simulink model "rapros_quadrotor_PID"  (R2013a)
settings: Solver=ode45  StartTime=0.0  StopTime=350  RelTol=1e-3
InitFcn:
  | parameters
values from neighbouring files (symbols this model uses):
  MATRIX = [-0.25 0 0.5 0.25 ... (first row only)    [parameters.m]
  X0 = [0;0;0;0;0;0;0;0;0;0;0;0]    [parameters.m]
libraries: instrumentlib x2, simulink x1
settings Model: Creator=root  LastModifiedBy=root
settings SolverCC: MaxConsecutiveMinStep=50000  AutoInsertRateTranBlk=on
settings DataIOCC: SignalLoggingSaveFormat=ModelDataLogs  SaveOutput=off  SaveTime=off
settings OptimizationCC: InlineParams=on  InlineInvariantSignals=on  StateBitsets=on  DataBitsets=on  UseTempVars=on  ZeroExternalMemoryAtStartup=off  ZeroInternalMemoryAtStartup=off  NoFixptDivByZeroProtection=on  OptimizeModelRefInitCode=on  LifeSpan=1
settings DebuggingCC: MultiTaskDSMMsg=warning  MultiTaskCondExecSysMsg=none  StrictBusMsg=None
settings HardwareCC: ProdIntDivRoundTo=Floor  ProdEndianess=LittleEndian  ProdHWDeviceType=Generic->Custom
settings RTWCC: SystemTargetFile=ert.tlc  TLCOptions=-p0  GenCodeOnly=on  TemplateMakefile=ert_default_tmf  Description=Embedded Coder  GenerateReport=on  RTWVerbose=off  ProcessScript=ert_make_rtw_hook  IncludeHyperlinkInReport=on  LaunchReport=on  IncludeERTFirstTime=on
settings CodeAppCC: ForceParamTrailComments=on  IgnoreCustomStorageClasses=off  SimulinkDataObjDesc=on  CustomSymbolStrGlobalVar=rt$N$M  CustomSymbolStrType=$N$M  CustomSymbolStrFcn=$N$M$F  CustomSymbolStrMacro=$N$M  InsertBlockDesc=on
settings ERTTargetCC: CodeReplacementLibrary=None  IncludeMdlTerminateFcn=off  SuppressErrorStatus=on  SupportAbsoluteTime=off  SupportNonFinite=off  SupportComplex=off  PurelyIntegerCode=on  RootIOFormat=Structure reference  ERTCustomFileTemplate=example_file_process.tlc

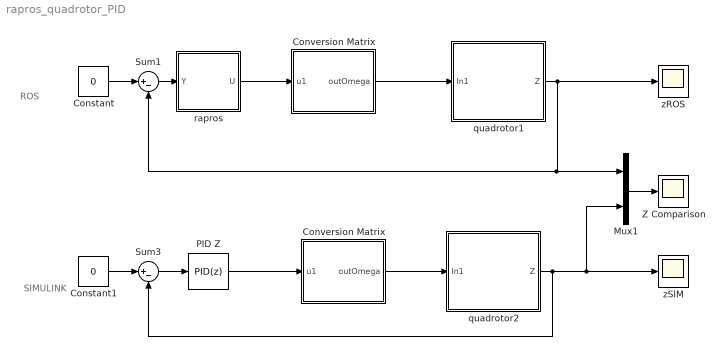
== system rapros_quadrotor_PID ==
  note: ROS
  note: SIMULINK
  Constant : Constant  Value=0
  Constant1 : Constant  Value=0
  Conversion Matrix : Subsystem
  "Conversion Matrix " : Subsystem
  Mux1 : Mux  Inputs=2
  PID Z : simulink/Continuous/PID Controller  Controller=PID  TimeDomain=Discrete-time  SampleTime=0.1  IntegratorMethod=Backward Euler  FilterMethod=Backward Euler  Form=Parallel  P=-22.9524857040326  I=-0.366329627958056  D=-215.804435520502  N=6.32298167776928  InitialConditionSource=internal  InitialConditionForIntegrator=0  InitialConditionForFilter=0  ExternalReset=none  LimitOutput=off  UpperSaturationLimit=inf  LowerSaturationLimit=-inf  LinearizeAsGain=off  AntiWindupMode=none  Kb=1  TrackingMode=off  Kt=1  PParamMin=[]  PParamMax=[]  IParamMin=[]  IParamMax=[]  DParamMin=[]  DParamMax=[]  NParamMin=[]  NParamMax=[]  KbParamMin=[]  KbParamMax=[]  KtParamMin=[]  KtParamMax=[]  POutMin=[]  POutMax=[]  IOutMin=[]  IOutMax=[]  DOutMin=[]  DOutMax=[]  NOutMin=[]  NOutMax=[]  KbOutMin=[]  KbOutMax=[]  KtOutMin=[]  KtOutMax=[]  IntegratorOutMin=[]  IntegratorOutMax=[]  FilterOutMin=[]  FilterOutMax=[]  SumOutMin=[]  SumOutMax=[]  SumI1OutMin=[]  SumI1OutMax=[]  SumI2OutMin=[]  SumI2OutMax=[]  SumI3OutMin=[]  SumI3OutMax=[]  SumDOutMin=[]  SumDOutMax=[]  SaturationOutMin=[]  SaturationOutMax=[]  IntegratorContinuousStateAttributes=''  IntegratorStateMustResolveToSignalObject=off  IntegratorRTWStateStorageClass=Auto  FilterContinuousStateAttributes=''  FilterStateMustResolveToSignalObject=off  FilterRTWStateStorageClass=Auto
  Sum1 : Sum  Inputs=|+-
  Sum3 : Sum  Inputs=|+-
  Z Comparison : Scope
      settings: YMin=17  YMax=31
  quadrotor1 : Subsystem
  quadrotor2 : Subsystem
  rapros : Subsystem  mask{output_size=1, input_size=1, Ts=0.1, IP='192.168.10.53', IPs='192.168.10.53'}
      mask prompts: output_size "Input dimension"; input_size "Output dimension"; Ts "Sample Time"; IP "Host address receive"; IPs "Host address send"
      mask init:
      | sys = get_param(0,'CurrentSystem');
      | input_size=[input_size 1];
      | datasize= mat2str(input_size);
      | ts= mat2str(Ts);
      | ip=IP;
      | Ip= mat2str(ip);
      | ips=IPs;
      | Ips= mat2str(ips);
      | set_param([sys '/rapros/Receive'],'DataSize',datasize);
      | set_param([sys '/rapros/Receive'],'Host',ip);
      | set_param([sys '/rapros/Receive'],'SampleTime',ts);
      | set_param([sys '/rapros/Send'],'Host',ips);
  zROS : Scope
      settings: YMin=24  YMax=31
  zSIM : Scope
      settings: SaveName=ScopeData2
  wires:
  "Conversion Matrix "/1(outOmega) -> quadrotor2/1(In1)
  PID Z/1 -> "Conversion Matrix "/1(u1)
  Mux1/1 -> Z Comparison/1
  Sum1/1 -> rapros/1(Y)
  Constant/1 -> Sum1/1
  quadrotor2/1(Z) -> Sum3/2, zSIM/1, Mux1/2
  Sum3/1 -> PID Z/1
  Constant1/1 -> Sum3/1
  quadrotor1/1(Z) -> zROS/1, Mux1/1, Sum1/2
  rapros/1(U) -> Conversion Matrix/1(u1)
  Conversion Matrix/1(outOmega) -> quadrotor1/1(In1)

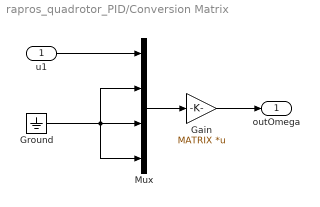
== system rapros_quadrotor_PID/Conversion Matrix ==
  u1 : Inport
  Gain : Gain  Gain=MATRIX  Multiplication=Matrix(K*u) (u vector)
  Ground : Ground
  Mux : Mux
  outOmega : Outport
  wires:
  u1/1 -> Mux/1
  Mux/1 -> Gain/1
  Gain/1 -> outOmega/1
  Ground/1 -> Mux/4, Mux/2, Mux/3

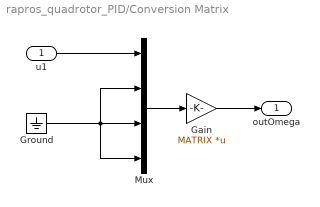
== system rapros_quadrotor_PID/Conversion Matrix  ==
  u1 : Inport
  Gain : Gain  Gain=MATRIX  Multiplication=Matrix(K*u) (u vector)
  Ground : Ground
  Mux : Mux
  outOmega : Outport
  wires:
  u1/1 -> Mux/1
  Mux/1 -> Gain/1
  Gain/1 -> outOmega/1
  Ground/1 -> Mux/4, Mux/2, Mux/3

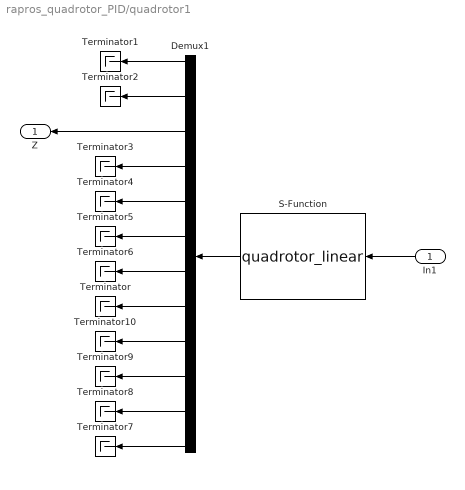
== system rapros_quadrotor_PID/quadrotor1 ==
  In1 : Inport
  Demux1 : Demux  Outputs=12
  S-Function : S-Function  FunctionName=quadrotor_linear  Parameters=X0(1),X0(2),X0(3),X0(4),X0(5),X0(6),X0(7),X0(8),X0(9),X0(10),X0(11),X0(12)  EnableBusSupport=off
  Terminator{,1..10} (11 alike) : Terminator
  Z : Outport
  wires:
  S-Function/1 -> Demux1/1
  In1/1 -> S-Function/1
  Demux1/12 -> Terminator7/1
  Demux1/4 -> Terminator3/1
  Demux1/6 -> Terminator5/1
  Demux1/5 -> Terminator4/1
  Demux1/11 -> Terminator8/1
  Demux1/10 -> Terminator9/1
  Demux1/9 -> Terminator10/1
  Demux1/8 -> Terminator/1
  Demux1/2 -> Terminator2/1
  Demux1/3 -> Z/1
  Demux1/7 -> Terminator6/1
  Demux1/1 -> Terminator1/1

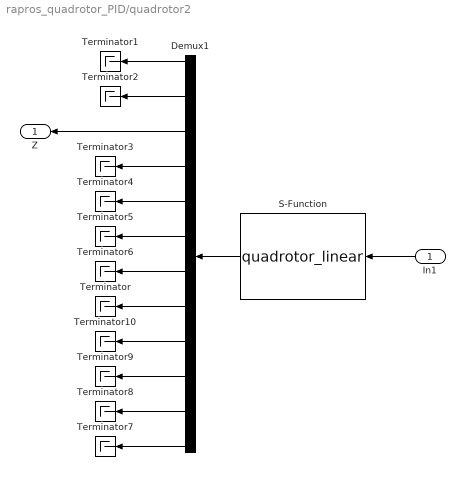
== system rapros_quadrotor_PID/quadrotor2 ==
  In1 : Inport
  Demux1 : Demux  Outputs=12
  S-Function : S-Function  FunctionName=quadrotor_linear  Parameters=X0(1),X0(2),X0(3),X0(4),X0(5),X0(6),X0(7),X0(8),X0(9),X0(10),X0(11),X0(12)  EnableBusSupport=off
  Terminator{,1..10} (11 alike) : Terminator
  Z : Outport
  wires:
  S-Function/1 -> Demux1/1
  In1/1 -> S-Function/1
  Demux1/12 -> Terminator7/1
  Demux1/4 -> Terminator3/1
  Demux1/6 -> Terminator5/1
  Demux1/5 -> Terminator4/1
  Demux1/11 -> Terminator8/1
  Demux1/10 -> Terminator9/1
  Demux1/9 -> Terminator10/1
  Demux1/8 -> Terminator/1
  Demux1/2 -> Terminator2/1
  Demux1/3 -> Z/1
  Demux1/7 -> Terminator6/1
  Demux1/1 -> Terminator1/1

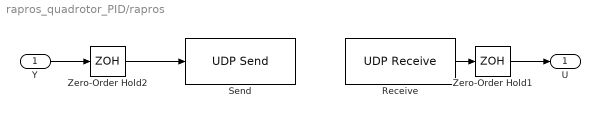
== system rapros_quadrotor_PID/rapros ==
  Y : Inport  PortDimensions=output_size
  Receive : instrumentlib/UDP Receive  Priority=2  Host=192.168.10.53  Port=25000  LocalPort=667  DataSize=[1 1]  EnableBlockingMode=on  Timeout=1  SampleTime=0.1  DataType=double  ByteOrder=LittleEndian
  Send : instrumentlib/UDP Send  Priority=1  Host=192.168.10.53  Port=25001  LocalPort=666  EnableBlockingMode=on  ByteOrder=LittleEndian
  Zero-Order Hold1 : ZeroOrderHold  SampleTime=Ts
  Zero-Order Hold2 : ZeroOrderHold  SampleTime=Ts
  U : Outport
  wires:
  Y/1 -> Zero-Order Hold2/1
  Zero-Order Hold2/1 -> Send/1
  Zero-Order Hold1/1 -> U/1
  Receive/1 -> Zero-Order Hold1/1
